simulink model "ProcessModelLittleRobot"  (R2014a)
settings: Solver=FixedStepDiscrete  StartTime=0.0  StopTime=15  FixedStep=0.05  RelTol=1e-3
PreLoadFcn:
  | SampleTime = 0.05;
undefined symbols (not defined in the file): DiscIntNeverNeededParam
settings Model: Creator=georg  LastModifiedBy=georg

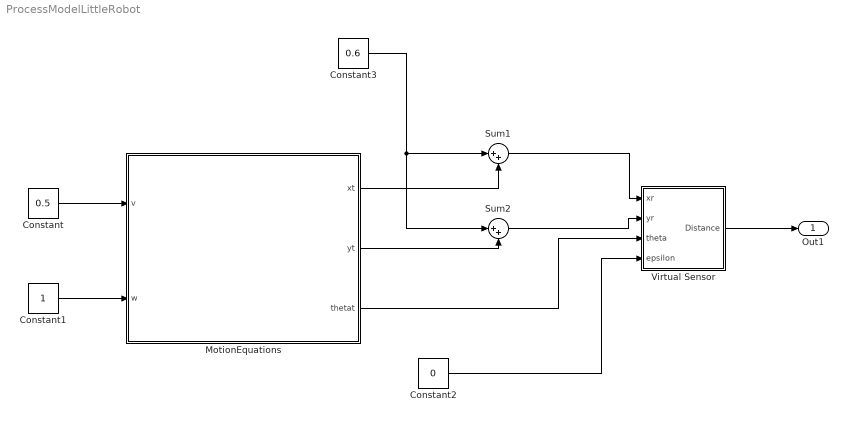
== system ProcessModelLittleRobot ==
  Constant : Constant  Value=0.5
  Constant1 : Constant
  Constant2 : Constant  Value=0
  Constant3 : Constant  Value=0.6
  MotionEquations : Subsystem
  Sum1 : Sum  Inputs=|++
  Sum2 : Sum  Inputs=|++
  Virtual Sensor : Subsystem
  Out1 : Outport
  wires:
  Constant/1 -> MotionEquations/1(v)
  Constant1/1 -> MotionEquations/2(w)
  Constant2/1 -> Virtual Sensor/4(epsilon)
  MotionEquations/1(xt) -> Sum1/2
  Constant3/1 -> Sum2/1, Sum1/1
  MotionEquations/2(yt) -> Sum2/2
  Sum1/1 -> Virtual Sensor/1(xr)
  Sum2/1 -> Virtual Sensor/2(yr)
  MotionEquations/3(thetat) -> Virtual Sensor/3(theta)
  Virtual Sensor/1(Distance) -> Out1/1

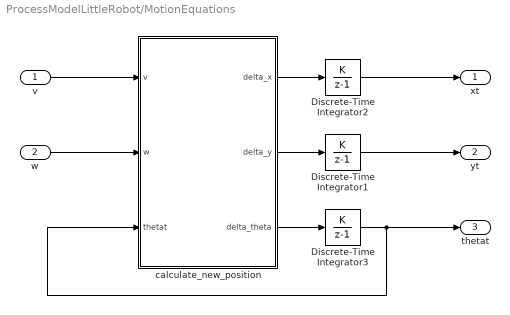
== system ProcessModelLittleRobot/MotionEquations ==
  v : Inport
  w : Inport  Port=2
  Discrete-Time Integrator1 : DiscreteIntegrator  IntegratorMethod=Accumulation: Forward Euler  SampleTime=-1  ICPrevOutput=DiscIntNeverNeededParam  ICPrevScaledInput=DiscIntNeverNeededParam
  Discrete-Time Integrator2 : DiscreteIntegrator  IntegratorMethod=Accumulation: Forward Euler  SampleTime=-1  ICPrevOutput=DiscIntNeverNeededParam  ICPrevScaledInput=DiscIntNeverNeededParam
  Discrete-Time Integrator3 : DiscreteIntegrator  IntegratorMethod=Accumulation: Forward Euler  SampleTime=-1  ICPrevOutput=DiscIntNeverNeededParam  ICPrevScaledInput=DiscIntNeverNeededParam
  calculate_new_position : Subsystem
  xt : Outport
  yt : Outport  Port=2
  thetat : Outport  Port=3
  wires:
  w/1 -> calculate_new_position/2(w)
  Discrete-Time Integrator1/1 -> yt/1
  v/1 -> calculate_new_position/1(v)
  calculate_new_position/3(delta_theta) -> Discrete-Time Integrator3/1
  Discrete-Time Integrator2/1 -> xt/1
  calculate_new_position/2(delta_y) -> Discrete-Time Integrator1/1
  calculate_new_position/1(delta_x) -> Discrete-Time Integrator2/1
  Discrete-Time Integrator3/1 -> calculate_new_position/3(thetat), thetat/1

== system ProcessModelLittleRobot/Virtual Sensor ==
  xr : Inport
  yr : Inport  Port=2
  theta : Inport  Port=3
  epsilon : Inport  Port=4
  Calculate Distance : Subsystem
  Sum : Sum  Inputs=|++
  Distance : Outport
  wires:
  Calculate Distance/1(x') -> Distance/1
  yr/1 -> Calculate Distance/2(yr)
  xr/1 -> Calculate Distance/1(xr)
  theta/1 -> Sum/1
  Sum/1 -> Calculate Distance/3(theta)
  epsilon/1 -> Sum/2

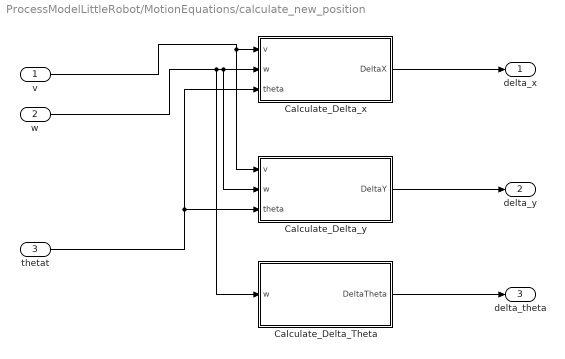
== system ProcessModelLittleRobot/MotionEquations/calculate_new_position ==
  v : Inport
  w : Inport  Port=2
  thetat : Inport  Port=3
  Calculate_Delta_Theta : Subsystem
  Calculate_Delta_x : Subsystem
  Calculate_Delta_y : Subsystem
  delta_x : Outport
  delta_y : Outport  Port=2
  delta_theta : Outport  Port=3
  wires:
  Calculate_Delta_y/1(DeltaY) -> delta_y/1
  Calculate_Delta_Theta/1(DeltaTheta) -> delta_theta/1
  Calculate_Delta_x/1(DeltaX) -> delta_x/1
  w/1 -> Calculate_Delta_y/2(w), Calculate_Delta_x/2(w), Calculate_Delta_Theta/1(w)
  thetat/1 -> Calculate_Delta_x/3(theta), Calculate_Delta_y/3(theta)
  v/1 -> Calculate_Delta_y/1(v), Calculate_Delta_x/1(v)

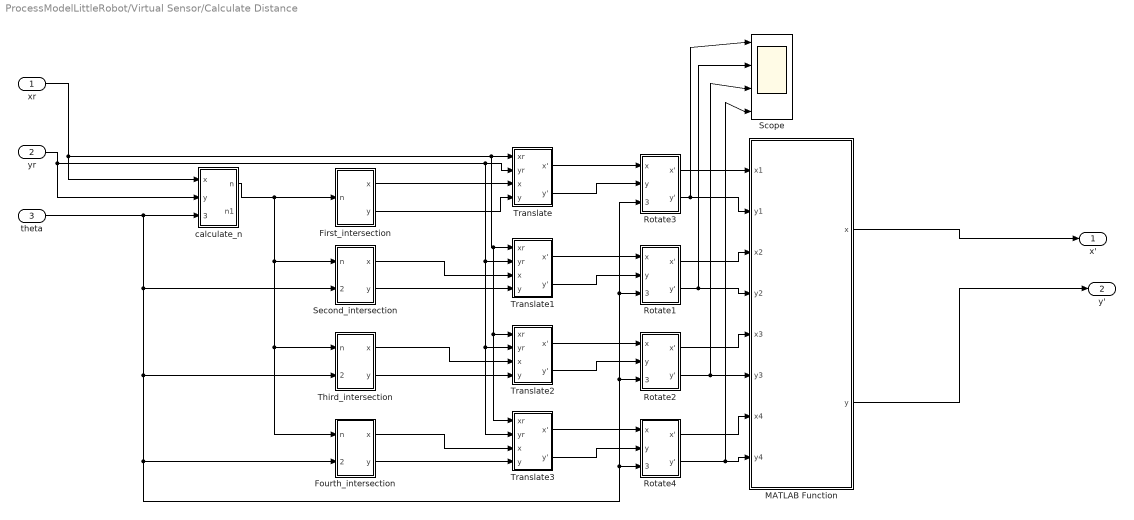
== system ProcessModelLittleRobot/Virtual Sensor/Calculate Distance ==
  xr : Inport
  yr : Inport  Port=2
  theta : Inport  Port=3
  First_intersection : Subsystem
  Fourth_intersection : Subsystem
  MATLAB Function : MATLAB Function  TreatAsAtomicUnit=on
  Rotate1 : Subsystem
  Rotate2 : Subsystem
  Rotate3 : Subsystem
  Rotate4 : Subsystem
  Scope : Scope  NumInputPorts=4
      settings: YMin=-5~-5~-5~-5  YMax=5~5~5~5  SaveName=ScopeData2
  Second_intersection : Subsystem
  Third_intersection : Subsystem
  Translate : Subsystem
  Translate1 : Subsystem
  Translate2 : Subsystem
  Translate3 : Subsystem
  calculate_n : Subsystem
  x' : Outport
  y' : Outport  Port=2
  wires:
  xr/1 -> calculate_n/1(x), Translate3/1(xr), Translate2/1(xr), Translate1/1(xr), Translate/1(xr)
  theta/1 -> Second_intersection/2(theta'), Third_intersection/2(theta'), Fourth_intersection/2(theta'), Rotate4/3(theta'), Rotate2/3(theta'), Rotate1/3(theta'), Rotate3/3(theta'), calculate_n/3(theta')
  calculate_n/1(n) -> Fourth_intersection/1(n), Third_intersection/1(n), Second_intersection/1(n), First_intersection/1(n)
  First_intersection/1(x) -> Translate/3(x)
  First_intersection/2(y) -> Translate/4(y)
  Second_intersection/1(x) -> Translate1/3(x)
  Second_intersection/2(y) -> Translate1/4(y)
  Third_intersection/2(y) -> Translate2/4(y)
  Third_intersection/1(x) -> Translate2/3(x)
  Fourth_intersection/2(y) -> Translate3/4(y)
  Fourth_intersection/1(x) -> Translate3/3(x)
  Translate3/2(y') -> Rotate4/2(y)
  Translate3/1(x') -> Rotate4/1(x)
  Translate2/1(x') -> Rotate2/1(x)
  Translate2/2(y') -> Rotate2/2(y)
  Translate1/1(x') -> Rotate1/1(x)
  Translate1/2(y') -> Rotate1/2(y)
  Translate/1(x') -> Rotate3/1(x)
  Translate/2(y') -> Rotate3/2(y)
  Rotate3/1(x') -> MATLAB Function/1(x1)
  Rotate1/1(x') -> MATLAB Function/3(x2)
  Rotate1/2(y') -> Scope/2, MATLAB Function/4(y2)
  Rotate2/1(x') -> MATLAB Function/5(x3)
  Rotate2/2(y') -> Scope/3, MATLAB Function/6(y3)
  Rotate4/1(x') -> MATLAB Function/7(x4)
  Rotate4/2(y') -> Scope/4, MATLAB Function/8(y4)
  MATLAB Function/1(x) -> x'/1
  MATLAB Function/2(y) -> y'/1
  yr/1 -> calculate_n/2(y), Translate3/2(yr), Translate2/2(yr), Translate1/2(yr), Translate/2(yr)
  Rotate3/2(y') -> Scope/1, MATLAB Function/2(y1)

== system ProcessModelLittleRobot/MotionEquations/calculate_new_position/Calculate_Delta_Theta ==
  w : Inport
  Gain : Gain  Gain=SampleTime
  DeltaTheta : Outport
  wires:
  w/1 -> Gain/1
  Gain/1 -> DeltaTheta/1

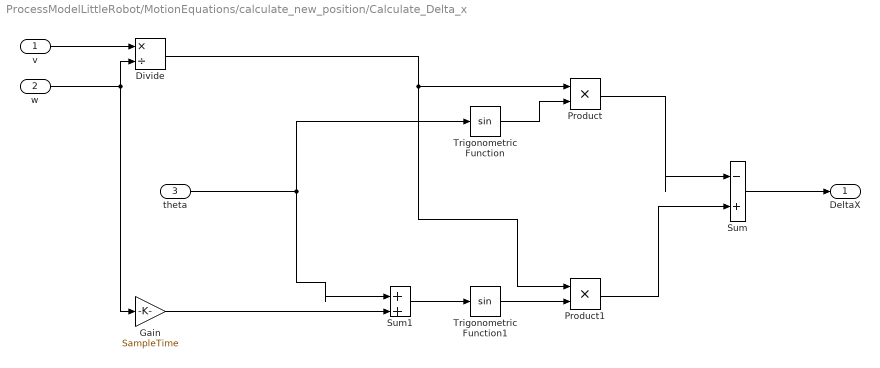
== system ProcessModelLittleRobot/MotionEquations/calculate_new_position/Calculate_Delta_x ==
  v : Inport
  w : Inport  Port=2
  theta : Inport  Port=3
  Divide : Product  Inputs=*/
  Gain : Gain  Gain=SampleTime
  Product : Product
  Product1 : Product
  Sum : Sum  Inputs=|-+
  Sum1 : Sum  Inputs=|++
  Trigonometric Function : Trigonometry
  Trigonometric Function1 : Trigonometry
  DeltaX : Outport
  wires:
  Trigonometric Function1/1 -> Product1/2
  Product/1 -> Sum/1
  Trigonometric Function/1 -> Product/2
  w/1 -> Gain/1, Divide/2
  v/1 -> Divide/1
  Divide/1 -> Product1/1, Product/1
  Gain/1 -> Sum1/2
  Product1/1 -> Sum/2
  Sum/1 -> DeltaX/1
  theta/1 -> Trigonometric Function/1, Sum1/1
  Sum1/1 -> Trigonometric Function1/1

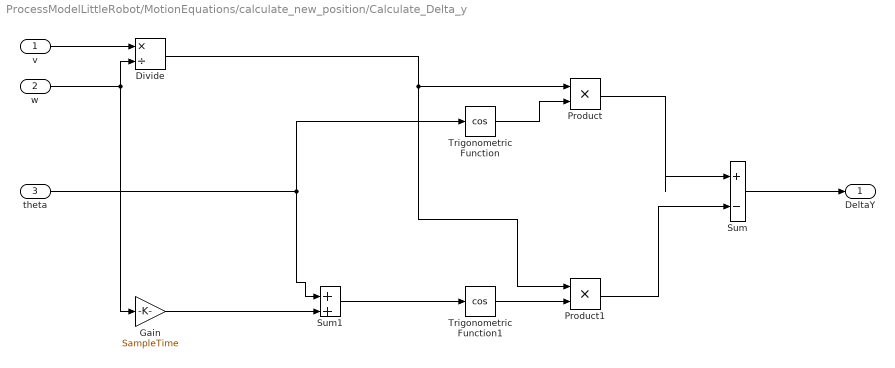
== system ProcessModelLittleRobot/MotionEquations/calculate_new_position/Calculate_Delta_y ==
  v : Inport
  w : Inport  Port=2
  theta : Inport  Port=3
  Divide : Product  Inputs=*/
  Gain : Gain  Gain=SampleTime
  Product : Product
  Product1 : Product
  Sum : Sum  Inputs=|+-
  Sum1 : Sum  Inputs=|++
  Trigonometric Function : Trigonometry  Operator=cos
  Trigonometric Function1 : Trigonometry  Operator=cos
  DeltaY : Outport
  wires:
  Trigonometric Function1/1 -> Product1/2
  theta/1 -> Trigonometric Function/1, Sum1/1
  Sum1/1 -> Trigonometric Function1/1
  Product/1 -> Sum/1
  Sum/1 -> DeltaY/1
  Trigonometric Function/1 -> Product/2
  w/1 -> Gain/1, Divide/2
  v/1 -> Divide/1
  Divide/1 -> Product1/1, Product/1
  Gain/1 -> Sum1/2
  Product1/1 -> Sum/2

== system ProcessModelLittleRobot/Virtual Sensor/Calculate Distance/First_intersection ==
  n : Inport
  zero : Constant  Value=0
  x : Outport
  y : Outport  Port=2
  wires:
  zero/1 -> x/1
  n/1 -> y/1

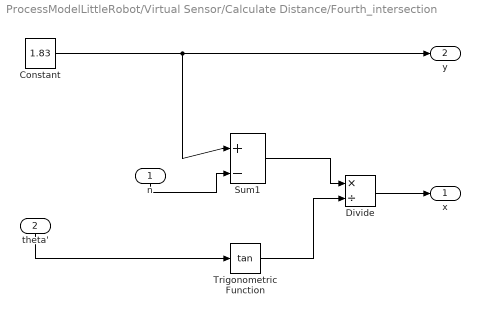
== system ProcessModelLittleRobot/Virtual Sensor/Calculate Distance/Fourth_intersection ==
  n : Inport
  theta' : Inport  Port=2
  Constant : Constant  Value=1.83
  Divide : Product  Inputs=*/
  Sum1 : Sum  Inputs=|+-
  Trigonometric Function : Trigonometry  Operator=tan
  x : Outport
  y : Outport  Port=2
  wires:
  Sum1/1 -> Divide/1
  theta'/1 -> Trigonometric Function/1
  Trigonometric Function/1 -> Divide/2
  Divide/1 -> x/1
  n/1 -> Sum1/2
  Constant/1 -> Sum1/1, y/1

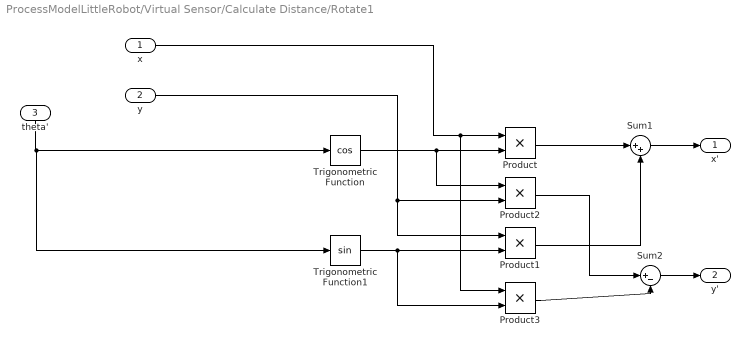
== system ProcessModelLittleRobot/Virtual Sensor/Calculate Distance/Rotate1 ==
  x : Inport
  y : Inport  Port=2
  theta' : Inport  Port=3
  Product{,1..3} (4 alike) : Product
  Sum1 : Sum  Inputs=|++
  Sum2 : Sum  Inputs=|+-
  Trigonometric Function : Trigonometry  Operator=cos
  Trigonometric Function1 : Trigonometry
  x' : Outport
  y' : Outport  Port=2
  wires:
  Product/1 -> Sum1/1
  Product1/1 -> Sum1/2
  x/1 -> Product3/1, Product/1
  Product2/1 -> Sum2/1
  Sum2/1 -> y'/1
  Sum1/1 -> x'/1
  Trigonometric Function/1 -> Product2/1, Product/2
  Product3/1 -> Sum2/2
  y/1 -> Product2/2, Product1/1
  Trigonometric Function1/1 -> Product3/2, Product1/2
  theta'/1 -> Trigonometric Function1/1, Trigonometric Function/1

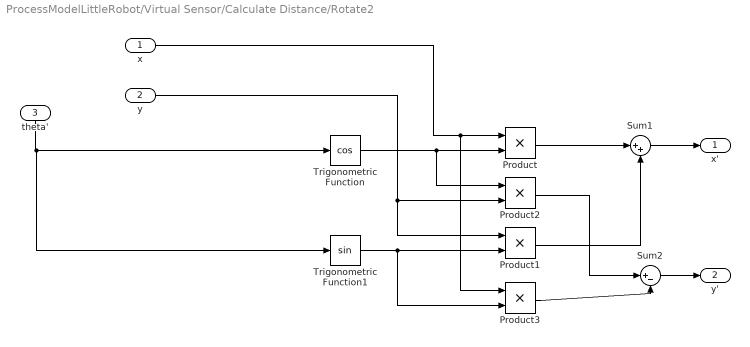
== system ProcessModelLittleRobot/Virtual Sensor/Calculate Distance/Rotate2 ==
  x : Inport
  y : Inport  Port=2
  theta' : Inport  Port=3
  Product{,1..3} (4 alike) : Product
  Sum1 : Sum  Inputs=|++
  Sum2 : Sum  Inputs=|+-
  Trigonometric Function : Trigonometry  Operator=cos
  Trigonometric Function1 : Trigonometry
  x' : Outport
  y' : Outport  Port=2
  wires:
  Product/1 -> Sum1/1
  Product1/1 -> Sum1/2
  x/1 -> Product3/1, Product/1
  Product2/1 -> Sum2/1
  Sum2/1 -> y'/1
  Sum1/1 -> x'/1
  Trigonometric Function/1 -> Product2/1, Product/2
  Product3/1 -> Sum2/2
  y/1 -> Product2/2, Product1/1
  Trigonometric Function1/1 -> Product3/2, Product1/2
  theta'/1 -> Trigonometric Function1/1, Trigonometric Function/1

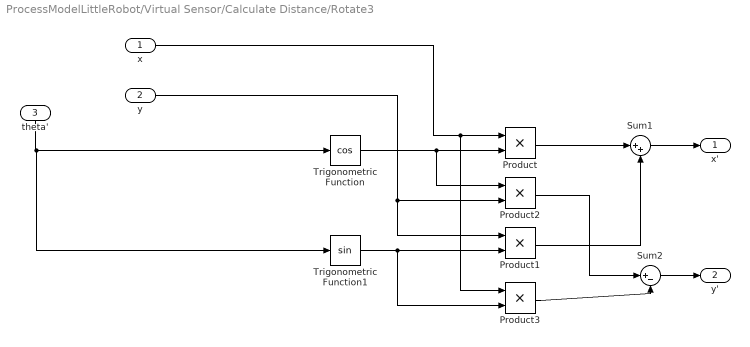
== system ProcessModelLittleRobot/Virtual Sensor/Calculate Distance/Rotate3 ==
  x : Inport
  y : Inport  Port=2
  theta' : Inport  Port=3
  Product{,1..3} (4 alike) : Product
  Sum1 : Sum  Inputs=|++
  Sum2 : Sum  Inputs=|+-
  Trigonometric Function : Trigonometry  Operator=cos
  Trigonometric Function1 : Trigonometry
  x' : Outport
  y' : Outport  Port=2
  wires:
  Product/1 -> Sum1/1
  Product1/1 -> Sum1/2
  x/1 -> Product3/1, Product/1
  Product2/1 -> Sum2/1
  Sum2/1 -> y'/1
  Sum1/1 -> x'/1
  Trigonometric Function/1 -> Product2/1, Product/2
  Product3/1 -> Sum2/2
  y/1 -> Product2/2, Product1/1
  Trigonometric Function1/1 -> Product3/2, Product1/2
  theta'/1 -> Trigonometric Function1/1, Trigonometric Function/1

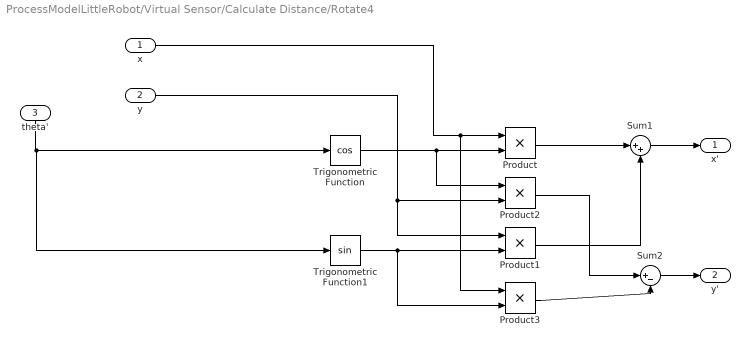
== system ProcessModelLittleRobot/Virtual Sensor/Calculate Distance/Rotate4 ==
  x : Inport
  y : Inport  Port=2
  theta' : Inport  Port=3
  Product{,1..3} (4 alike) : Product
  Sum1 : Sum  Inputs=|++
  Sum2 : Sum  Inputs=|+-
  Trigonometric Function : Trigonometry  Operator=cos
  Trigonometric Function1 : Trigonometry
  x' : Outport
  y' : Outport  Port=2
  wires:
  Product/1 -> Sum1/1
  Product1/1 -> Sum1/2
  x/1 -> Product3/1, Product/1
  Product2/1 -> Sum2/1
  Sum2/1 -> y'/1
  Sum1/1 -> x'/1
  Trigonometric Function/1 -> Product2/1, Product/2
  Product3/1 -> Sum2/2
  y/1 -> Product2/2, Product1/1
  Trigonometric Function1/1 -> Product3/2, Product1/2
  theta'/1 -> Trigonometric Function1/1, Trigonometric Function/1

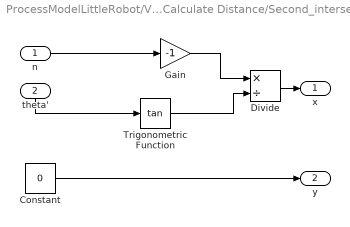
== system ProcessModelLittleRobot/Virtual Sensor/Calculate Distance/Second_intersection ==
  n : Inport
  theta' : Inport  Port=2
  Constant : Constant  Value=0
  Divide : Product  Inputs=*/
  Gain : Gain  Gain=-1
  Trigonometric Function : Trigonometry  Operator=tan
  x : Outport
  y : Outport  Port=2
  wires:
  Trigonometric Function/1 -> Divide/2
  Gain/1 -> Divide/1
  n/1 -> Gain/1
  Divide/1 -> x/1
  theta'/1 -> Trigonometric Function/1
  Constant/1 -> y/1

== system ProcessModelLittleRobot/Virtual Sensor/Calculate Distance/Third_intersection ==
  n : Inport
  theta' : Inport  Port=2
  Constant : Constant  Value=1.22
  Product : Product
  Sum1 : Sum  Inputs=|++
  Trigonometric Function : Trigonometry  Operator=tan
  x : Outport
  y : Outport  Port=2
  wires:
  n/1 -> Sum1/1
  Sum1/1 -> y/1
  theta'/1 -> Trigonometric Function/1
  Product/1 -> Sum1/2
  Trigonometric Function/1 -> Product/2
  Constant/1 -> Product/1, x/1

== system ProcessModelLittleRobot/Virtual Sensor/Calculate Distance/Translate ==
  xr : Inport
  yr : Inport  Port=2
  x : Inport  Port=3
  y : Inport  Port=4
  Add : Sum  Inputs=-+
  Add1 : Sum  Inputs=-+
  x' : Outport
  y' : Outport  Port=2
  wires:
  y/1 -> Add1/2
  yr/1 -> Add1/1
  x/1 -> Add/2
  Add/1 -> x'/1
  xr/1 -> Add/1
  Add1/1 -> y'/1

== system ProcessModelLittleRobot/Virtual Sensor/Calculate Distance/Translate1 ==
  xr : Inport
  yr : Inport  Port=2
  x : Inport  Port=3
  y : Inport  Port=4
  Add : Sum  Inputs=-+
  Add1 : Sum  Inputs=-+
  x' : Outport
  y' : Outport  Port=2
  wires:
  y/1 -> Add1/2
  yr/1 -> Add1/1
  x/1 -> Add/2
  Add/1 -> x'/1
  xr/1 -> Add/1
  Add1/1 -> y'/1

== system ProcessModelLittleRobot/Virtual Sensor/Calculate Distance/Translate2 ==
  xr : Inport
  yr : Inport  Port=2
  x : Inport  Port=3
  y : Inport  Port=4
  Add : Sum  Inputs=-+
  Add1 : Sum  Inputs=-+
  x' : Outport
  y' : Outport  Port=2
  wires:
  y/1 -> Add1/2
  yr/1 -> Add1/1
  x/1 -> Add/2
  Add/1 -> x'/1
  xr/1 -> Add/1
  Add1/1 -> y'/1

== system ProcessModelLittleRobot/Virtual Sensor/Calculate Distance/Translate3 ==
  xr : Inport
  yr : Inport  Port=2
  x : Inport  Port=3
  y : Inport  Port=4
  Add : Sum  Inputs=-+
  Add1 : Sum  Inputs=-+
  x' : Outport
  y' : Outport  Port=2
  wires:
  y/1 -> Add1/2
  yr/1 -> Add1/1
  x/1 -> Add/2
  Add/1 -> x'/1
  xr/1 -> Add/1
  Add1/1 -> y'/1

== system ProcessModelLittleRobot/Virtual Sensor/Calculate Distance/calculate_n ==
  x : Inport
  y : Inport  Port=2
  theta' : Inport  Port=3
  Product : Product
  Sum1 : Sum  Inputs=|+-
  Trigonometric Function : Trigonometry  Operator=tan
  n : Outport
  n1 : Outport  Port=2
  wires:
  Product/1 -> Sum1/2
  theta'/1 -> Trigonometric Function/1
  x/1 -> Product/1
  Trigonometric Function/1 -> n1/1, Product/2
  y/1 -> Sum1/1
  Sum1/1 -> n/1

== matlab function ProcessModelLittleRobot/Virtual Sensor/Calculate Distance/MATLAB Function ==
  data: x output; x1 input; y1 input; y output; x2 input; y2 input; x3 input; y3 input; x4 input; y4 input
function [x,y] = fcn(x1,y1,x2,y2,x3,y3,x4,y4)

zx1 = 0;
zy1 = 0;
zx2 = 0;
zy2 = 0;
cnt = 1;

if(x1 > 0)
    if(cnt == 1)
        zx1 = x1;
        zy1 = y1;
        cnt = cnt + 1;
    else
        if(cnt == 2)
            zx2 = x1;
            zy2 = y1;
            cnt = cnt + 1;
        end
    end
        
end

if(x2 > 0)
    if(cnt == 1)
        zx1 = x2;
        zy1 = y2;
        cnt = cnt + 1;
    else
        if(cnt == 2)
            zx2 = x2;
            zy2 = y2;
            cnt = cnt + 1;
        end
    end
        
end

if(x3 > 0)
    if(cnt == 1)
        zx1 = x3;
        zy1 = y3;
        cnt = cnt + 1;
    else
        if(cnt == 2)
            zx2 = x3;
            zy2 = y3;
            cnt = cnt + 1;
        end
    end
        
end


if(x4 > 0)
    if(cnt == 1)
        zx1 = x4;
        zy1 = y4;
        cnt = cnt + 1;
    else
        if(cnt == 2)
            zx2 = x4;
            zy2 = y4;
            cnt = cnt + 1;
        end
    end
        
end

if(zx1<zx2)
    x = zx1;
    y = zy1;
else
    x = zx2;
    y = zy2;
end

end
